simulink model "OM1"  (R2019b)
settings: Solver=VariableStepAuto  StartTime=0.0  StopTime=t_final  MaxStep=0.001  RelTol=1e-3
values from neighbouring files (symbols this model uses):
  K1 = 1 + 0.1*(2*rand()-1)    [PI_regul.m]
  K2 = 1 + 0.1*(2*rand()-1)    [PI_regul.m]
  Ki = Kia*T0    [PI_regul.m]
  Kia = 1/(2*Tu*Kob)    [PI_regul.m]
  Kp = Kpa    [PI_regul.m]
  Kpa = T1/(2*Tu*Kob)    [PI_regul.m]
  st = 0    [PI_regul.m]
  T0 = 0.1    [PI_regul.m]
  T1 = 1 + 0.1*(2*rand()-1)    [PI_regul.m]
  T2 = 0.2 + 0.1*(2*rand()-1)    [PI_regul.m]
  Tzap = T0/2    (= 0.05)    [PI_regul.m]
settings Model: Creator=Anton Mayorov  LastModifiedBy=bedla
settings DataIOCC: ReturnWorkspaceOutputs=off
settings DebuggingCC: ArithmeticOperatorsInVariantConditions=warning
settings SFSimCC: SimUseLocalCustomCode=off  CustomCodeUndefinedFunction=UseInterfaceOnly
settings RTWCC: RTWUseLocalCustomCode=off

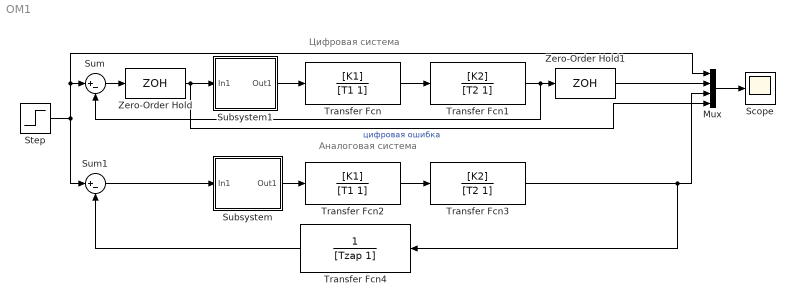
== system OM1 ==
  note: Аналоговая система
  note: Цифровая система
  Mux : Mux
  Scope : Scope
  Step : Step  Time=st  SampleTime=0
  Subsystem : Subsystem
  Subsystem1 : Subsystem
  Sum : Sum  Inputs=|+-
  Sum1 : Sum  Inputs=|+-
  Transfer Fcn : TransferFcn  Numerator=[K1]  Denominator=[T1 1]
  Transfer Fcn1 : TransferFcn  Numerator=[K2]  Denominator=[T2 1]
  Transfer Fcn2 : TransferFcn  Numerator=[K1]  Denominator=[T1 1]
  Transfer Fcn3 : TransferFcn  Numerator=[K2]  Denominator=[T2 1]
  Transfer Fcn4 : TransferFcn  Denominator=[Tzap 1]
  Zero-Order Hold : ZeroOrderHold  SampleTime=T0
  Zero-Order Hold1 : ZeroOrderHold  SampleTime=T0
  wires:
  Zero-Order Hold/1 -> Subsystem1/1(In1), Mux/4  "цифровая ошибка"
  Transfer Fcn/1 -> Transfer Fcn1/1
  Mux/1 -> Scope/1
  Subsystem1/1(Out1) -> Transfer Fcn/1
  Transfer Fcn1/1 -> Sum/2, Zero-Order Hold1/1
  Sum/1 -> Zero-Order Hold/1
  Step/1 -> Mux/1, Sum/1, Sum1/1
  Sum1/1 -> Subsystem/1(In1)
  Transfer Fcn3/1 -> Mux/3, Transfer Fcn4/1
  Subsystem/1(Out1) -> Transfer Fcn2/1
  Transfer Fcn2/1 -> Transfer Fcn3/1
  Zero-Order Hold1/1 -> Mux/2
  Transfer Fcn4/1 -> Sum1/2

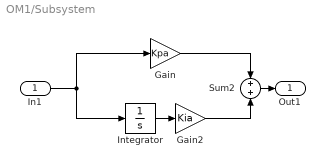
== system OM1/Subsystem ==
  In1 : Inport
  Gain : Gain  Gain=Kpa
  Gain2 : Gain  Gain=Kia
  Integrator : Integrator
  Sum2 : Sum
  Out1 : Outport
  wires:
  In1/1 -> Gain/1, Integrator/1
  Integrator/1 -> Gain2/1
  Gain/1 -> Sum2/1
  Sum2/1 -> Out1/1
  Gain2/1 -> Sum2/2

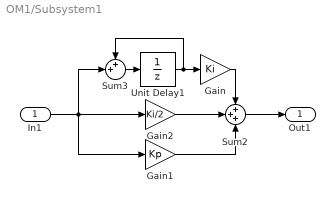
== system OM1/Subsystem1 ==
  In1 : Inport
  Gain : Gain  Gain=Ki
  Gain1 : Gain  Gain=Kp
  Gain2 : Gain  Gain=Ki/2
  Sum2 : Sum  Inputs=+++
  Sum3 : Sum  Inputs=++|
  Unit Delay1 : UnitDelay  SampleTime=-1  HasFrameUpgradeWarning=on
  Out1 : Outport
  wires:
  Sum3/1 -> Unit Delay1/1
  Unit Delay1/1 -> Gain/1, Sum3/1
  Gain/1 -> Sum2/1
  In1/1 -> Gain2/1, Gain1/1, Sum3/2
  Gain2/1 -> Sum2/2
  Sum2/1 -> Out1/1
  Gain1/1 -> Sum2/3
